simulink model "dynamic_vehicle"  (R2021b)
settings: Solver=VariableStepAuto  StartTime=0.0  StopTime=100  MaxStep=0.001  RelTol=1e-3
undefined symbols (not defined in the file or in its folder): D_inv, g, m, xbc, ybc
libraries: simulink x2
settings Model: Creator=A0072685  LastModifiedBy=A0072685

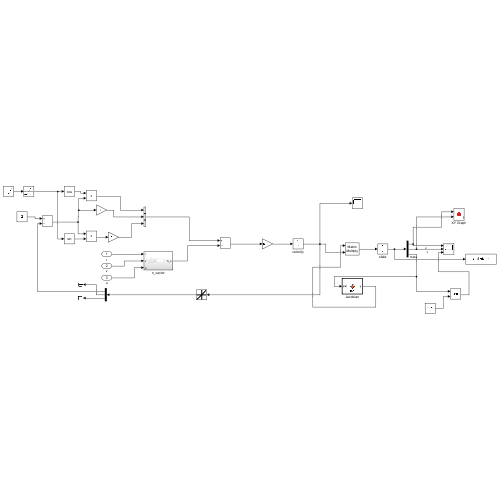
[thumbnail: Simulink's stored preview of the top-level diagram]
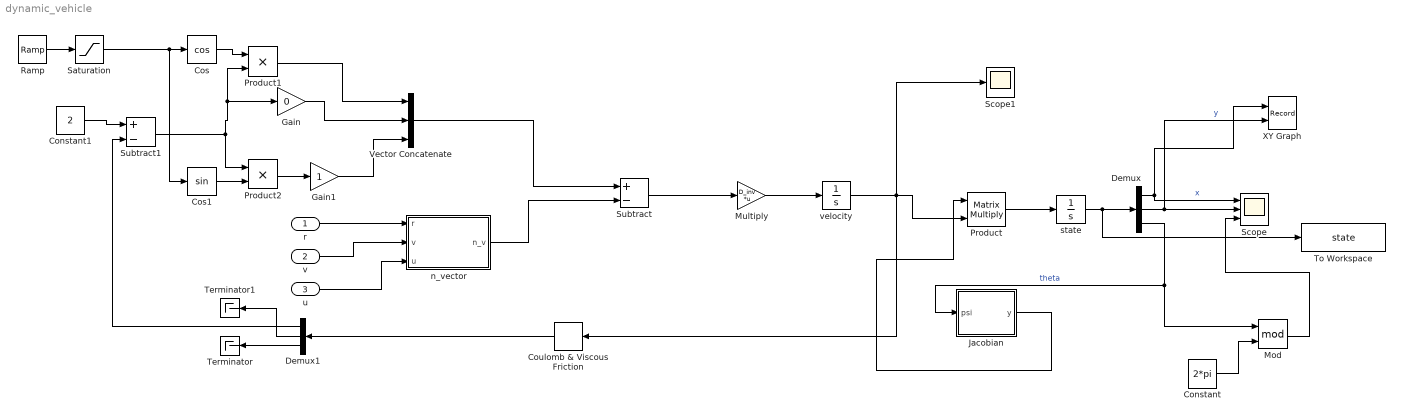
== system dynamic_vehicle ==
  r : Inport
  v : Inport  Port=2
  u : Inport  Port=3
  Constant : Constant  Value=2*pi
  Constant1 : Constant  Value=2
  Cos : Trigonometry  Operator=cos
  Cos1 : Trigonometry
  Coulomb & Viscous Friction : simulink/Discontinuities/Coulomb & Viscous Friction  offset=0  gain=0.02*m*g
  Demux : Demux  Outputs=3
  Demux1 : Demux  Outputs=3
  Gain : Gain  Gain=0
  Gain1 : Gain
  Jacobian : MATLAB Function  TreatAsAtomicUnit=on
  Mod : Math  Operator=mod  SaturateOnIntegerOverflow=on
  Multiply : Gain  Gain=D_inv  Multiplication=Matrix(K*u)
  Product : Product  Multiplication=Matrix(*)
  Product1 : Product
  Product2 : Product
  Ramp : simulink/Sources/Ramp  slope=0.01  start=0  InitialOutput=0
  Saturation : Saturate  UpperLimit=0.1  LowerLimit=-2
  Scope : Scope  NumInputPorts=3
  Scope1 : Scope
  Subtract : Sum  Inputs=+-
  Subtract1 : Sum  Inputs=+-
  Terminator : Terminator
  Terminator1 : Terminator
  To Workspace : ToWorkspace  VariableName=state  SaveFormat=Timeseries  SampleTime=-1
  Vector Concatenate : Concatenate  NumInputs=3
  XY Graph : Record  FileSettingsInternal="{\"entries\":[{\"content\":{\"excelSettings\":{\"content\":{},\"type\":\"Streamout.ExcelSettings\"}},\"type\":\"Streamout.FileSettingStorage\",\"uuid\":\"3e31ba68-2283-492e-a761-73db27a570a0\"}],\"packageUris\":[\"http://schema.mathworks.com/mf0/streamout_blocks/R2020a\"],\"version\":\"1.0\"}"  Layout=[1 1]  SignalsInternal="{\"entries\":[{\"content\":{\"signals\":[{\"content\":{\"blockPath\":[\"dynamic_vehicle/XY Graph\"],\"channel\":[],\"dimensions\":[1],\"domain\":\"dynamic_vehicle/XY Graph\",\"lineColor\":\"#a2142f\",\"plots\":[1],\"port\":1,\"sid\":[\"\"],\"signalID\":20,\"signalName\":\"x\"},\"type\":\"RecordBlkView.Signal\",\"uuid\":\"ea64e725-ad34-4bb1-a450-275d4804edac\"},{\"content\":{\"blockPath\":[\"dynamic_vehicle/XY Graph\"],\"channel\":[],\"dimensions\":[1],\"domain\":\"dynamic_vehicle/XY Graph\",\"lineColor\":\"#139fff\",\"plots\":[1],\"port\":2,\"sid\":[\"\"],\"signalID\":24,\"signalName\":\"y\"},\"type\":\"RecordBlkView.Signal\",\"uuid\":\"c08974b2-6e12-48da-ad09-676d99a5e03e\"}]},\"type\":\"RecordBlkView.InputSignals\",\"uuid\":\"6d612a72-e1c5-418c-af46-babfbc759e20\"}],\"packageUris\":[\"http://schema.mathworks.com/mf0/streamout_blocks/R2020a\"],\"version\":\"1.0\"}"  VisualizationBindings="{\"xyplotplugin\":{\"info\":[{\"series\":[{\"bindingParametersList\":[{\"parameter\":\"X-Axis\",\"signalID\":20,\"signalName\":\"x\"},{\"parameter\":\"Y-Axis\",\"signalID\":24,\"signalName\":\"y\"}],\"seriesID\":41695}],\"subplotID\":1}]}}"  CompatibilityTag=XY  st=-1
  n_vector : Subsystem
  state : Integrator
  velocity : Integrator  InitialCondition=[0.01,0,0]
  wires:
  r/1 -> n_vector/1(r)
  v/1 -> n_vector/2(v)
  u/1 -> n_vector/3(u)
  Vector Concatenate/1 -> Subtract/1
  n_vector/1(n_v) -> Subtract/2
  Multiply/1 -> velocity/1
  Jacobian/1(y) -> Product/1
  Product/1 -> state/1
  state/1 -> To Workspace/1, Demux/1
  Demux/3 -> Mod/1, Jacobian/1(psi)  "theta"
  Demux/1 -> XY Graph/1, Scope/1  "x"
  Demux/2 -> XY Graph/2, Scope/2  "y"
  Saturation/1 -> Cos1/1, Cos/1
  Cos/1 -> Product1/1
  Product1/1 -> Vector Concatenate/1
  Gain/1 -> Vector Concatenate/2
  Cos1/1 -> Product2/2
  Product2/1 -> Gain1/1
  Gain1/1 -> Vector Concatenate/3
  Ramp/1 -> Saturation/1
  Constant/1 -> Mod/2
  Mod/1 -> Scope/3
  Subtract/1 -> Multiply/1
  velocity/1 -> Coulomb & Viscous Friction/1, Scope1/1, Product/2
  Constant1/1 -> Subtract1/1
  Subtract1/1 -> Product1/2, Gain/1, Product2/1
  Coulomb & Viscous Friction/1 -> Demux1/1
  Demux1/1 -> Subtract1/2
  Demux1/2 -> Terminator1/1
  Demux1/3 -> Terminator/1

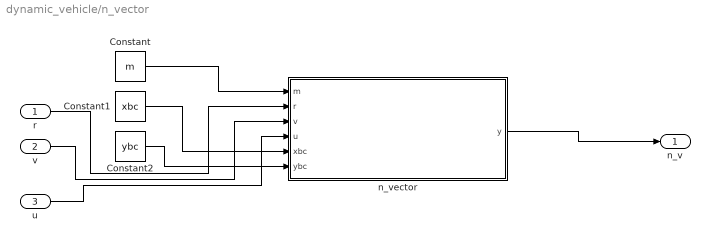
== system dynamic_vehicle/n_vector ==
  r : Inport
  v : Inport  Port=2
  u : Inport  Port=3
  Constant : Constant  Value=m
  Constant1 : Constant  Value=xbc
  Constant2 : Constant  Value=ybc
  n_vector : MATLAB Function  TreatAsAtomicUnit=on
  n_v : Outport
  wires:
  v/1 -> n_vector/3(v)
  Constant2/1 -> n_vector/6(ybc)
  Constant/1 -> n_vector/1(m)
  r/1 -> n_vector/2(r)
  u/1 -> n_vector/4(u)
  n_vector/1(y) -> n_v/1
  Constant1/1 -> n_vector/5(xbc)

== matlab function dynamic_vehicle/Jacobian ==
  data: psi input; y output
function y = fcn(psi)
%#codegen
    J_eta = [cos(psi), -sin(psi), 0 ; 
             sin(psi), cos(psi),  0 ; 
             0 , 0 , 1];  % Jacobian

y = J_eta;

== matlab function dynamic_vehicle/n_vector/n_vector ==
  data: m input; r input; v input; u input; y output; xbc input; ybc input
function y = fcn(m,r,v,u, xbc, ybc)
%#codegen
n_v = [-m*r*(v+xbc*r);
        m*r*(u-ybc*r);
        m*r*(xbc*u-ybc*v)];

y = n_v;
